simulink model "Code_Gen_Model"  (R2023b)
settings: Solver=FixedStepDiscrete  StartTime=0.0  StopTime=inf  FixedStep=t_sample  RelTol=1e-3
settings Model: Creator=FIRSTMentor  LastModifiedBy=ander
settings OptimizationCC: DefaultParameterBehavior=Inlined  StrengthReduction=on  PassReuseOutputArgsAs=Individual arguments  ZeroExternalMemoryAtStartup=off  ZeroInternalMemoryAtStartup=off  OptimizeBlockOrder=speed  OptimizationPriority=Speed  OptimizationCustomize=off  MultiThreadedLoops=on  EfficientTunableParamExpr=on
settings DebuggingCC: MergeDetectMultiDrivingBlocksExec=none  ParameterTunabilityLossMsg=error
settings HardwareCC: ProdBitPerPointer=32  ProdBitPerSizeT=32  ProdBitPerPtrDiffT=32  ProdLargestAtomicInteger=Long  ProdWordSize=32  ProdHWDeviceType=ARM Compatible->ARM 7
settings ModelReferenceCC: PropagateSignalLabelsOutOfModel=off
settings SFSimCC: MATLABDynamicMemAlloc=off
settings RTWCC: Description=Embedded Coder  SystemTargetFile=ert.tlc  GenCodeOnly=on  TemplateMakefile=ert_default_tmf  Toolchain=MinGW64 | gmake (64-bit Windows)
settings CodeAppCC: ForceParamTrailComments=on  IgnoreCustomStorageClasses=off  OperatorAnnotations=on  SimulinkDataObjDesc=on  SFDataObjDesc=on  InsertBlockDesc=on
settings ERTTargetCC: TargetLangStandard=C99 (ISO)  SupportVariableSizeSignals=on  ParenthesesLevel=Maximum  InlinedParameterPlacement=NonHierarchical  ERTCustomFileTemplate=example_file_process.tlc

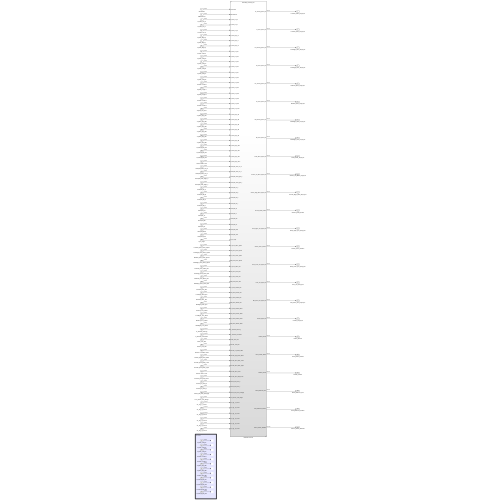
[thumbnail: Simulink's stored preview of the top-level diagram]
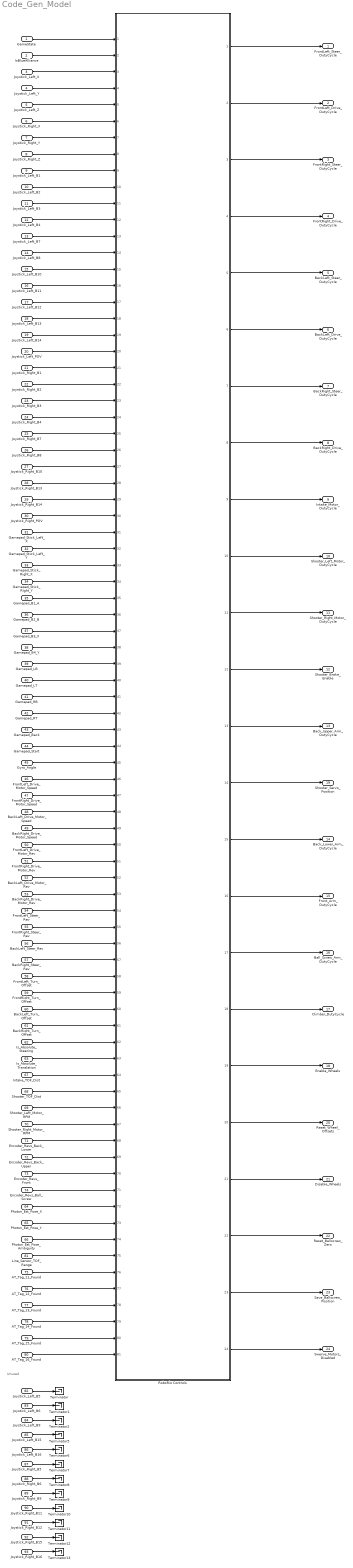
== system Code_Gen_Model ==
  note: Unused
  GameState : Inport
  IsBlueAlliance : Inport  Port=2
  Joystick_Left_X : Inport  Port=3
  Joystick_Left_Y : Inport  Port=4
  Joystick_Left_Z : Inport  Port=5
  Joystick_Right_X : Inport  Port=6
  Joystick_Right_Y : Inport  Port=7
  Joystick_Right_Z : Inport  Port=8
  Joystick_Left_B1 : Inport  Port=9
  Joystick_Left_B2 : Inport  Port=10
  Joystick_Left_B3 : Inport  Port=11
  Joystick_Left_B4 : Inport  Port=12
  Joystick_Left_B7 : Inport  Port=13
  Joystick_Left_B8 : Inport  Port=14
  Joystick_Left_B10 : Inport  Port=15
  Joystick_Left_B11 : Inport  Port=16
  Joystick_Left_B12 : Inport  Port=17
  Joystick_Left_B13 : Inport  Port=18
  Joystick_Left_B14 : Inport  Port=19
  Joystick_Left_POV : Inport  Port=20
  Joystick_Right_B1 : Inport  Port=21
  Joystick_Right_B2 : Inport  Port=22
  Joystick_Right_B3 : Inport  Port=23
  Joystick_Right_B4 : Inport  Port=24
  Joystick_Right_B7 : Inport  Port=25
  Joystick_Right_B8 : Inport  Port=26
  Joystick_Right_B10 : Inport  Port=27
  Joystick_Right_B13 : Inport  Port=28
  Joystick_Right_B14 : Inport  Port=29
  Joystick_Right_POV : Inport  Port=30
  Gamepad_Stick_Left_X : Inport  Port=31
  Gamepad_Stick_Left_Y : Inport  Port=32
  Gamepad_Stick_Right_X : Inport  Port=33
  Gamepad_Stick_Right_Y : Inport  Port=34
  Gamepad_B1_A : Inport  Port=35
  Gamepad_B2_B : Inport  Port=36
  Gamepad_B3_X : Inport  Port=37
  Gamepad_B4_Y : Inport  Port=38
  Gamepad_LB : Inport  Port=39
  Gamepad_LT : Inport  Port=40
  Gamepad_RB : Inport  Port=41
  Gamepad_RT : Inport  Port=42
  Gamepad_Back : Inport  Port=43
  Gamepad_Start : Inport  Port=44
  Gyro_Angle : Inport  Port=45
  FrontLeft_Drive_Motor_Speed : Inport  Port=46
  FrontRight_Drive_Motor_Speed : Inport  Port=47
  BackLeft_Drive_Motor_Speed : Inport  Port=48
  BackRight_Drive_Motor_Speed : Inport  Port=49
  FrontLeft_Drive_Motor_Rev : Inport  Port=50
  FrontRight_Drive_Motor_Rev : Inport  Port=51
  BackLeft_Drive_Motor_Rev : Inport  Port=52
  BackRight_Drive_Motor_Rev : Inport  Port=53
  FrontLeft_Steer_Rev : Inport  Port=54
  FrontRight_Steer_Rev : Inport  Port=55
  BackLeft_Steer_Rev : Inport  Port=56
  BackRight_Steer_Rev : Inport  Port=57
  FrontLeft_Turn_Offset : Inport  Port=58
  FrontRight_Turn_Offset : Inport  Port=59
  BackLeft_Turn_Offset : Inport  Port=60
  BackRight_Turn_Offset : Inport  Port=61
  Is_Absolute_Steering : Inport  Port=62
  Is_Absolute_Translation : Inport  Port=63
  Photon_Est_Pose_X : Inport  Port=64
  Photon_Est_Pose_Y : Inport  Port=65
  Photon_Est_Pose_Ambiguity : Inport  Port=66
  Intake_TOF_Dist : Inport  Port=67
  Shooter_TOF_Dist : Inport  Port=68
  Shooter_Left_Motor_RPM : Inport  Port=69
  Shooter_Right_Motor_RPM : Inport  Port=70
  Encoder_Revs_Back_Lower : Inport  Port=71
  Encoder_Revs_Back_Upper : Inport  Port=72
  Encoder_Revs_Front : Inport  Port=73
  Encoder_Revs_Ball_Screw : Inport  Port=74
  AT_Tag_11_Found : Inport  Port=75
  AT_Tag_12_Found : Inport  Port=76
  AT_Tag_13_Found : Inport  Port=77
  AT_Tag_14_Found : Inport  Port=78
  AT_Tag_15_Found : Inport  Port=79
  AT_Tag_16_Found : Inport  Port=80
  Line_Sensor_TOF_Range : Inport  Port=81
  Joystick_Left_B5 : Inport  Port=82
  Joystick_Left_B6 : Inport  Port=83
  Joystick_Left_B9 : Inport  Port=84
  Joystick_Left_B15 : Inport  Port=85
  Joystick_Left_B16 : Inport  Port=86
  Joystick_Right_B5 : Inport  Port=87
  Joystick_Right_B6 : Inport  Port=88
  Joystick_Right_B9 : Inport  Port=89
  Joystick_Right_B11 : Inport  Port=90
  Joystick_Right_B12 : Inport  Port=91
  Joystick_Right_B15 : Inport  Port=92
  Joystick_Right_B16 : Inport  Port=93
  RoboRio Controls : Subsystem  ReferencedSubsystem=RoboRio_Controls_sub
  Terminator{,1..2,5..13} (12 alike) : Terminator
  FrontLeft_Steer_DutyCycle : Outport
  FrontLeft_Drive_DutyCycle : Outport  Port=2
  FrontRight_Steer_DutyCycle : Outport  Port=3
  FrontRight_Drive_DutyCycle : Outport  Port=4
  BackLeft_Steer_DutyCycle : Outport  Port=5
  BackLeft_Drive_DutyCycle : Outport  Port=6
  BackRight_Steer_DutyCycle : Outport  Port=7
  BackRight_Drive_DutyCycle : Outport  Port=8
  Intake_Motor_DutyCycle : Outport  Port=9
  Shooter_Left_Motor_DutyCycle : Outport  Port=10
  Shooter_Right_Motor_DutyCycle : Outport  Port=11
  Shooter_Brake_Enable : Outport  Port=12
  Back_Upper_Arm_DutyCycle : Outport  Port=13
  Back_Lower_Arm_DutyCycle : Outport  Port=14
  Front_Arm_DutyCycle : Outport  Port=15
  Ball_Screw_Arm_DutyCycle : Outport  Port=16
  Climber_DutyCycle : Outport  Port=17
  Enable_Wheels : Outport  Port=18
  Shooter_Servo_Position : Outport  Port=19
  Reset_Wheel_Offsets : Outport  Port=20
  Disable_Wheels : Outport  Port=21
  Reset_Ballscrew_Zero : Outport  Port=22
  Save_Ballscrew_Position : Outport  Port=23
  Swerve_Motors_Disabled : Outport  Port=24
  wires:
  Joystick_Right_B10/1 -> RoboRio Controls/27
  Joystick_Right_B8/1 -> RoboRio Controls/26
  Joystick_Right_B7/1 -> RoboRio Controls/25
  Joystick_Right_B12/1 -> Terminator11/1
  Joystick_Right_B4/1 -> RoboRio Controls/24
  GameState/1 -> RoboRio Controls/1
  RoboRio Controls/8 -> BackRight_Drive_DutyCycle/1
  Joystick_Right_B15/1 -> Terminator12/1
  Joystick_Left_B15/1 -> Terminator5/1
  Joystick_Right_B5/1 -> Terminator7/1
  Joystick_Right_B6/1 -> Terminator8/1
  RoboRio Controls/16 -> Front_Arm_DutyCycle/1
  Joystick_Left_B6/1 -> Terminator1/1
  Joystick_Left_B5/1 -> Terminator/1
  Joystick_Left_B16/1 -> Terminator6/1
  Gamepad_Stick_Left_X/1 -> RoboRio Controls/31
  Joystick_Right_POV/1 -> RoboRio Controls/30
  Joystick_Right_B14/1 -> RoboRio Controls/29
  Joystick_Right_B13/1 -> RoboRio Controls/28
  Joystick_Left_B9/1 -> Terminator2/1
  Joystick_Right_B3/1 -> RoboRio Controls/23
  Joystick_Right_B2/1 -> RoboRio Controls/22
  Joystick_Right_B1/1 -> RoboRio Controls/21
  Joystick_Left_POV/1 -> RoboRio Controls/20
  Joystick_Right_B11/1 -> Terminator10/1
  Joystick_Right_B9/1 -> Terminator9/1
  Joystick_Right_B16/1 -> Terminator13/1
  Photon_Est_Pose_Y/1 -> RoboRio Controls/73
  Joystick_Left_Z/1 -> RoboRio Controls/5
  Encoder_Revs_Ball_Screw/1 -> RoboRio Controls/71
  Joystick_Left_Y/1 -> RoboRio Controls/4
  Joystick_Left_X/1 -> RoboRio Controls/3
  IsBlueAlliance/1 -> RoboRio Controls/2
  Gamepad_B2_B/1 -> RoboRio Controls/36
  AT_Tag_16_Found/1 -> RoboRio Controls/81
  Joystick_Left_B1/1 -> RoboRio Controls/9
  AT_Tag_14_Found/1 -> RoboRio Controls/79
  Joystick_Right_Z/1 -> RoboRio Controls/8
  RoboRio Controls/3 -> FrontRight_Steer_DutyCycle/1
  Joystick_Right_Y/1 -> RoboRio Controls/7
  Joystick_Right_X/1 -> RoboRio Controls/6
  BackRight_Steer_Rev/1 -> RoboRio Controls/57
  Joystick_Left_B7/1 -> RoboRio Controls/13
  FrontRight_Steer_Rev/1 -> RoboRio Controls/55
  Joystick_Left_B4/1 -> RoboRio Controls/12
  Joystick_Left_B3/1 -> RoboRio Controls/11
  Joystick_Left_B2/1 -> RoboRio Controls/10
  Shooter_TOF_Dist/1 -> RoboRio Controls/65
  Joystick_Left_B14/1 -> RoboRio Controls/19
  Is_Absolute_Translation/1 -> RoboRio Controls/63
  Joystick_Left_B13/1 -> RoboRio Controls/18
  Joystick_Left_B10/1 -> RoboRio Controls/15
  Joystick_Left_B8/1 -> RoboRio Controls/14
  Joystick_Left_B11/1 -> RoboRio Controls/16
  Joystick_Left_B12/1 -> RoboRio Controls/17
  Gamepad_B1_A/1 -> RoboRio Controls/35
  RoboRio Controls/1 -> FrontLeft_Steer_DutyCycle/1
  Gamepad_Stick_Right_Y/1 -> RoboRio Controls/34
  Gamepad_Stick_Right_X/1 -> RoboRio Controls/33
  Gamepad_Stick_Left_Y/1 -> RoboRio Controls/32
  Gamepad_B3_X/1 -> RoboRio Controls/37
  Gamepad_RB/1 -> RoboRio Controls/41
  Gamepad_LT/1 -> RoboRio Controls/40
  Gamepad_LB/1 -> RoboRio Controls/39
  Gamepad_B4_Y/1 -> RoboRio Controls/38
  Gyro_Angle/1 -> RoboRio Controls/45
  Gamepad_Start/1 -> RoboRio Controls/44
  Gamepad_Back/1 -> RoboRio Controls/43
  RoboRio Controls/17 -> Ball_Screw_Arm_DutyCycle/1
  Gamepad_RT/1 -> RoboRio Controls/42
  BackRight_Drive_Motor_Speed/1 -> RoboRio Controls/49
  BackLeft_Drive_Motor_Speed/1 -> RoboRio Controls/48
  FrontRight_Drive_Motor_Speed/1 -> RoboRio Controls/47
  FrontLeft_Drive_Motor_Speed/1 -> RoboRio Controls/46
  RoboRio Controls/12 -> Shooter_Brake_Enable/1
  BackLeft_Drive_Motor_Rev/1 -> RoboRio Controls/52
  FrontRight_Drive_Motor_Rev/1 -> RoboRio Controls/51
  FrontLeft_Drive_Motor_Rev/1 -> RoboRio Controls/50
  BackRight_Drive_Motor_Rev/1 -> RoboRio Controls/53
  FrontLeft_Steer_Rev/1 -> RoboRio Controls/54
  BackLeft_Steer_Rev/1 -> RoboRio Controls/56
  FrontLeft_Turn_Offset/1 -> RoboRio Controls/58
  FrontRight_Turn_Offset/1 -> RoboRio Controls/59
  BackLeft_Turn_Offset/1 -> RoboRio Controls/60
  BackRight_Turn_Offset/1 -> RoboRio Controls/61
  Is_Absolute_Steering/1 -> RoboRio Controls/62
  Intake_TOF_Dist/1 -> RoboRio Controls/64
  Shooter_Left_Motor_RPM/1 -> RoboRio Controls/66
  Shooter_Right_Motor_RPM/1 -> RoboRio Controls/67
  Encoder_Revs_Back_Lower/1 -> RoboRio Controls/68
  Encoder_Revs_Back_Upper/1 -> RoboRio Controls/69
  Encoder_Revs_Front/1 -> RoboRio Controls/70
  Photon_Est_Pose_X/1 -> RoboRio Controls/72
  Photon_Est_Pose_Ambiguity/1 -> RoboRio Controls/74
  AT_Tag_11_Found/1 -> RoboRio Controls/76
  AT_Tag_12_Found/1 -> RoboRio Controls/77
  AT_Tag_13_Found/1 -> RoboRio Controls/78
  AT_Tag_15_Found/1 -> RoboRio Controls/80
  Line_Sensor_TOF_Range/1 -> RoboRio Controls/75
  RoboRio Controls/2 -> FrontLeft_Drive_DutyCycle/1
  RoboRio Controls/4 -> FrontRight_Drive_DutyCycle/1
  RoboRio Controls/6 -> BackLeft_Drive_DutyCycle/1
  RoboRio Controls/5 -> BackLeft_Steer_DutyCycle/1
  RoboRio Controls/7 -> BackRight_Steer_DutyCycle/1
  RoboRio Controls/9 -> Intake_Motor_DutyCycle/1
  RoboRio Controls/10 -> Shooter_Left_Motor_DutyCycle/1
  RoboRio Controls/11 -> Shooter_Right_Motor_DutyCycle/1
  RoboRio Controls/13 -> Back_Upper_Arm_DutyCycle/1
  RoboRio Controls/15 -> Back_Lower_Arm_DutyCycle/1
  RoboRio Controls/18 -> Climber_DutyCycle/1
  RoboRio Controls/14 -> Shooter_Servo_Position/1
  RoboRio Controls/23 -> Save_Ballscrew_Position/1
  RoboRio Controls/22 -> Reset_Ballscrew_Zero/1
  RoboRio Controls/21 -> Disable_Wheels/1
  RoboRio Controls/20 -> Reset_Wheel_Offsets/1
  RoboRio Controls/24 -> Swerve_Motors_Disabled/1
  RoboRio Controls/19 -> Enable_Wheels/1
